simulink model "collection_of_goodies"  (Simulink 5.0)
settings: Solver=ode45  StartTime=0.0  StopTime=10.0  RelTol=1e-3
values from neighbouring files (symbols this model uses):
  c = 4.4*tp/(pi*ts)    [PD_sketch_design.m]
  I = [Ixx,Ixy,Ixz;Iyx,Iyy,Iyz;Izx,Izy,Izz]    [starshotmath.m]
  q0 = [qmatlab(2:4),qmatlab(1)]'    [starshot_DC_KD_setup.m]    (also in starshot_DC_setup.m; temp.m)
  s = tf('s')    [starshot_DC_setup.m]
undefined symbols (not defined in the file or in its folder): a1_T_CMG, a2_T_CMG, a3_T_CMG, AccLim, b1_T_CMG, b2_T_CMG, b3_T_CMG, CFthreshoff, CFthreshon, filt1d, filt1n, filt2d, filt2n, filts1n, filts2d, filts2n, fine, h, h_cos_cmg, h_init, h_sin_cmg, hdmax, hmax, I34, Id, Igm1d, Igm1n, IgmAAFd, invI, invId, Is, Isat, IsatSp, k1_obs, k2_obs, Kt, Kts, lam, Lgm, ls, lt, M34, muE, Ngear, P0, pfd, pfn, q_init, r0, rc_ampl, rc_harm, rc_phase, Rgm, Smin, SmotDrag, spin_init, TachAAFd, TAU_ACS, tr_ampl, tr_harm ... (+8)
libraries: simulink x27, mblibv1 x3, dspinverses x1
(part 2 of 2)

== system collection_of_goodies/Kane Damper wbn is inertial body rate in body axes apply (-Tdamp) to rigid body/Cross1 ==
  A : Inport
  B : Inport  Port=2
  Mux4 : Mux  Inputs=3
  Product{,1..5} (6 alike) : Product  SaturateOnIntegerOverflow=on  InputSameDT=on
  Sum : Sum  Inputs=+-  SaturateOnIntegerOverflow=on  InputSameDT=on
  Sum1 : Sum  Inputs=+-  SaturateOnIntegerOverflow=on  InputSameDT=on
  Sum2 : Sum  Inputs=+-  SaturateOnIntegerOverflow=on  InputSameDT=on
  demux2 : Demux  Outputs=3
  demux3 : Demux  Outputs=3
  AxB : Outport  InitialOutput=0
  wires:
  Mux4/1 -> AxB/1
  Sum2/1 -> Mux4/3
  Sum1/1 -> Mux4/2
  Sum/1 -> Mux4/1
  Product5/1 -> Sum2/2
  Product4/1 -> Sum2/1
  Product3/1 -> Sum1/2
  Product2/1 -> Sum1/1
  Product1/1 -> Sum/2
  Product/1 -> Sum/1
  demux3/1 -> Product5/2, Product2/2
  demux2/2 -> Product5/1, Product/1
  demux3/2 -> Product4/2, Product1/2
  demux2/1 -> Product4/1, Product3/1
  demux3/3 -> Product3/2, Product/2
  demux2/3 -> Product2/1, Product1/1
  B/1 -> demux3/1
  A/1 -> demux2/1

== system collection_of_goodies/Orbit EOM/norm ==
  v : Inport
  Dot Product : simulink/Math Operations/Dot Product
  Math Function : Math  Operator=sqrt
  Saturation : Saturate  UpperLimit=1e20  LowerLimit=1e-10
  |v| : Outport
  wires:
  Saturation/1 -> |v|/1
  Math Function/1 -> Saturation/1
  Dot Product/1 -> Math Function/1
  v/1 -> Dot Product/2, Dot Product/1

== system collection_of_goodies/Propagate Attitude via DCM (not as nice as the quaternion method)/(a*phi)^X ==
  In1 : Inport
  3x3 : simulink/Math Operations/Reshape  OutputDimensionality=Customize  OutputDimensions=[3,3]
  Demux : Demux  Outputs=3
  Gain : Gain  Gain=-1  SaturateOnIntegerOverflow=on
  Gain1 : Gain  Gain=-1  SaturateOnIntegerOverflow=on
  Gain2 : Gain  Gain=-1  SaturateOnIntegerOverflow=on
  Mux : Mux  Inputs=9
  "diag 0 " : Constant  Value=0
  Out1 : Outport
  wires:
  In1/1 -> Demux/1
  3x3/1 -> Out1/1
  "diag 0 "/1 -> Mux/1, Mux/5, Mux/9
  Mux/1 -> 3x3/1
  Demux/3 -> Mux/2, Gain1/1
  Gain/1 -> Mux/3
  Demux/2 -> Gain/1, Mux/7
  Gain1/1 -> Mux/4
  Demux/1 -> Mux/6, Gain2/1
  Gain2/1 -> Mux/8

== system collection_of_goodies/Propagate Attitude via Quaternion/q_normalize ==
  q_in : Inport  PortDimensions=4
  Dot Product : simulink/Math Operations/Dot Product
  Math Function : Math  Operator=sqrt
  Product : Product  Inputs=*/  SaturateOnIntegerOverflow=on  InputSameDT=on
  q_out : Outport
  wires:
  q_in/1 -> Dot Product/1, Dot Product/2, Product/1
  Dot Product/1 -> Math Function/1
  Math Function/1 -> Product/2
  Product/1 -> q_out/1

== system collection_of_goodies/Propagate Attitude via Quaternion/quat_multiply ==
  q_bc : Inport
  q_ab : Inport  Port=2
  Mux : Mux  Inputs=2
  Mux1 : Mux
  qerr1 : Fcn  Expr=u(4)*u(5)+u(3)*u(6)-u(2)*u(7)+u(1)*u(8)
  qerr2 : Fcn  Expr=-u(3)*u(5)+u(4)*u(6)+u(1)*u(7)+u(2)*u(8)
  qerr3 : Fcn  Expr=u(2)*u(5)-u(1)*u(6)+u(4)*u(7)+u(3)*u(8)
  qerr4 : Fcn  Expr=-u(1)*u(5)-u(2)*u(6)-u(3)*u(7)+u(4)*u(8)
  q_ac : Outport
  wires:
  Mux1/1 -> q_ac/1
  qerr4/1 -> Mux1/4
  qerr3/1 -> Mux1/3
  qerr2/1 -> Mux1/2
  qerr1/1 -> Mux1/1
  Mux/1 -> qerr4/1, qerr3/1, qerr2/1, qerr1/1
  q_ab/1 -> Mux/2
  q_bc/1 -> Mux/1

== system collection_of_goodies/Quaternion Integration/q_normalize ==
  q_in : Inport  PortDimensions=4
  Dot Product : simulink/Math Operations/Dot Product
  Math Function : Math  Operator=sqrt
  Product : Product  Inputs=*/  SaturateOnIntegerOverflow=on  InputSameDT=on
  q_out : Outport
  wires:
  q_in/1 -> Dot Product/1, Dot Product/2, Product/1
  Dot Product/1 -> Math Function/1
  Math Function/1 -> Product/2
  Product/1 -> q_out/1

== system collection_of_goodies/Quaternion Integration/qderiv ==
  w : Inport
  q : Inport  Port=2
  Mux : Mux  Inputs=2
  Mux1 : Mux
  qd1 : Fcn  Expr=(u(7)*u(1)-u(6)*u(2)+u(5)*u(3))/2
  qd2 : Fcn  Expr=(u(6)*u(1)+u(7)*u(2)-u(4)*u(3))/2
  qd3 : Fcn  Expr=(-u(5)*u(1)+u(4)*u(2)+u(7)*u(3))/2
  qd4 : Fcn  Expr=(-u(4)*u(1)-u(5)*u(2)-u(6)*u(3))/2
  qd : Outport
  wires:
  w/1 -> Mux/1
  q/1 -> Mux/2
  Mux/1 -> qd1/1, qd2/1, qd3/1, qd4/1
  qd1/1 -> Mux1/1
  qd2/1 -> Mux1/2
  qd3/1 -> Mux1/3
  qd4/1 -> Mux1/4
  Mux1/1 -> qd/1

== system collection_of_goodies/Rigid Body with Momentum Actuators and energy dissipation/Cross ==
  A : Inport
  B : Inport  Port=2
  Mux4 : Mux  Inputs=3
  Product{,1..5} (6 alike) : Product  SaturateOnIntegerOverflow=on  InputSameDT=on
  Sum : Sum  Inputs=+-  SaturateOnIntegerOverflow=on  InputSameDT=on
  Sum1 : Sum  Inputs=+-  SaturateOnIntegerOverflow=on  InputSameDT=on
  Sum2 : Sum  Inputs=+-  SaturateOnIntegerOverflow=on  InputSameDT=on
  demux2 : Demux  Outputs=3
  demux3 : Demux  Outputs=3
  AxB : Outport  InitialOutput=0
  wires:
  Mux4/1 -> AxB/1
  Sum2/1 -> Mux4/3
  Sum1/1 -> Mux4/2
  Sum/1 -> Mux4/1
  Product5/1 -> Sum2/2
  Product4/1 -> Sum2/1
  Product3/1 -> Sum1/2
  Product2/1 -> Sum1/1
  Product1/1 -> Sum/2
  Product/1 -> Sum/1
  demux3/1 -> Product5/2, Product2/2
  demux2/2 -> Product5/1, Product/1
  demux3/2 -> Product4/2, Product1/2
  demux2/1 -> Product4/1, Product3/1
  demux3/3 -> Product3/2, Product/2
  demux2/3 -> Product2/1, Product1/1
  B/1 -> demux3/1
  A/1 -> demux2/1

== system collection_of_goodies/Rigid Body with Momentum Actuators and energy dissipation/Cross1 ==
  A : Inport
  B : Inport  Port=2
  Mux4 : Mux  Inputs=3
  Product{,1..5} (6 alike) : Product  SaturateOnIntegerOverflow=on  InputSameDT=on
  Sum : Sum  Inputs=+-  SaturateOnIntegerOverflow=on  InputSameDT=on
  Sum1 : Sum  Inputs=+-  SaturateOnIntegerOverflow=on  InputSameDT=on
  Sum2 : Sum  Inputs=+-  SaturateOnIntegerOverflow=on  InputSameDT=on
  demux2 : Demux  Outputs=3
  demux3 : Demux  Outputs=3
  AxB : Outport  InitialOutput=0
  wires:
  Mux4/1 -> AxB/1
  Sum2/1 -> Mux4/3
  Sum1/1 -> Mux4/2
  Sum/1 -> Mux4/1
  Product5/1 -> Sum2/2
  Product4/1 -> Sum2/1
  Product3/1 -> Sum1/2
  Product2/1 -> Sum1/1
  Product1/1 -> Sum/2
  Product/1 -> Sum/1
  demux3/1 -> Product5/2, Product2/2
  demux2/2 -> Product5/1, Product/1
  demux3/2 -> Product4/2, Product1/2
  demux2/1 -> Product4/1, Product3/1
  demux3/3 -> Product3/2, Product/2
  demux2/3 -> Product2/1, Product1/1
  B/1 -> demux3/1
  A/1 -> demux2/1

== system collection_of_goodies/Rigid Body with Momentum Actuators and energy dissipation/Quaternion Integration ==
  w_Body : Inport
  Integrator1 : Integrator  InitialCondition=q_init
  q_normalize : Subsystem
  qderiv : Subsystem
  q_I_Body : Outport
  wires:
  qderiv/1(qd) -> Integrator1/1
  Integrator1/1 -> q_normalize/1(q_in)
  q_normalize/1(q_out) -> q_I_Body/1, qderiv/2(q)
  w_Body/1 -> qderiv/1(w)

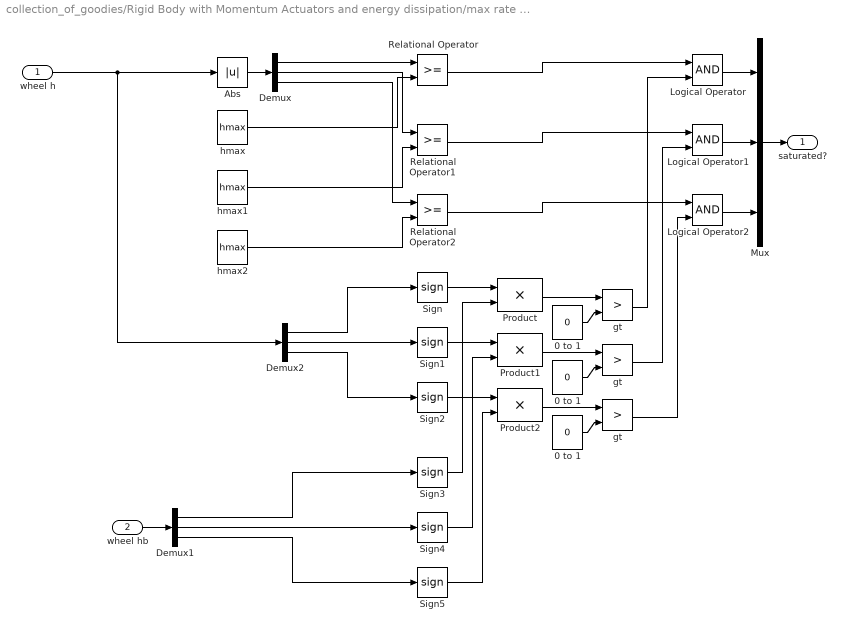
== system collection_of_goodies/Rigid Body with Momentum Actuators and energy dissipation/max rate check ==
  wheel h : Inport
  wheel hb : Inport  Port=2
  0 to 1 : Constant  Value=0  VectorParams1D=off
  "0 to 1 " : Constant  Value=0  VectorParams1D=off
  "0 to 1  " : Constant  Value=0  VectorParams1D=off
  Abs : Abs  SaturateOnIntegerOverflow=on
  Demux : Demux  Outputs=3
  Demux1 : Demux  Outputs=3
  Demux2 : Demux  Outputs=3
  Logical Operator : Logic
  Logical Operator1 : Logic
  Logical Operator2 : Logic
  Mux : Mux  Inputs=3
  Product : Product  SaturateOnIntegerOverflow=on  InputSameDT=on
  Product1 : Product  SaturateOnIntegerOverflow=on  InputSameDT=on
  Product2 : Product  SaturateOnIntegerOverflow=on  InputSameDT=on
  Relational Operator : RelationalOperator  InputSameDT=on
  Relational Operator1 : RelationalOperator  InputSameDT=on
  Relational Operator2 : RelationalOperator  InputSameDT=on
  Sign{,1..5} (6 alike) : Signum
  gt : RelationalOperator  Operator=>  InputSameDT=on
  "gt " : RelationalOperator  Operator=>  InputSameDT=on
  "gt  " : RelationalOperator  Operator=>  InputSameDT=on
  hmax : Constant  Value=hmax  VectorParams1D=off
  hmax1 : Constant  Value=hmax  VectorParams1D=off
  hmax2 : Constant  Value=hmax  VectorParams1D=off
  saturated? : Outport
  wires:
  Abs/1 -> Demux/1
  Demux/1 -> Relational Operator/1
  Demux/2 -> Relational Operator1/1
  Demux/3 -> Relational Operator2/1
  hmax/1 -> Relational Operator/2
  hmax1/1 -> Relational Operator1/2
  hmax2/1 -> Relational Operator2/2
  wheel h/1 -> Abs/1, Demux2/1
  Mux/1 -> saturated?/1
  wheel hb/1 -> Demux1/1
  Demux1/1 -> Sign3/1
  Demux1/2 -> Sign4/1
  Demux1/3 -> Sign5/1
  Sign/1 -> Product/1
  Sign3/1 -> Product/2
  Sign1/1 -> Product1/1
  Sign4/1 -> Product1/2
  Sign2/1 -> Product2/1
  Sign5/1 -> Product2/2
  0 to 1/1 -> gt/2
  Product/1 -> gt/1
  "0 to 1 "/1 -> "gt "/2
  Product1/1 -> "gt "/1
  "0 to 1  "/1 -> "gt  "/2
  Product2/1 -> "gt  "/1
  Logical Operator/1 -> Mux/1
  Logical Operator1/1 -> Mux/2
  Logical Operator2/1 -> Mux/3
  Relational Operator/1 -> Logical Operator/1
  Relational Operator1/1 -> Logical Operator1/1
  Relational Operator2/1 -> Logical Operator2/1
  gt/1 -> Logical Operator/2
  "gt "/1 -> Logical Operator1/2
  "gt  "/1 -> Logical Operator2/2
  Demux2/1 -> Sign/1
  Demux2/2 -> Sign1/1
  Demux2/3 -> Sign2/1

== system collection_of_goodies/SimMechanics embedded h body/cross2 ==
  a : Inport
  b : Inport  Port=2
  Demux : Demux  Outputs=3
  Demux1 : Demux  Outputs=3
  Fcn : Fcn  Expr=-u(3)*u(5)+u(2)*u(6)
  Fcn1 : Fcn  Expr=u(3)*u(4)-u(1)*u(6)
  Fcn2 : Fcn  Expr=-u(2)*u(4)+u(1)*u(5)
  Mux : Mux  Inputs=6
  Mux1 : Mux  Inputs=3
  a x b : Outport
  wires:
  Mux/1 -> Fcn/1, Fcn1/1, Fcn2/1
  Mux1/1 -> a x b/1
  Fcn/1 -> Mux1/1
  Fcn1/1 -> Mux1/2
  Fcn2/1 -> Mux1/3
  Demux/1 -> Mux/1
  Demux/2 -> Mux/2
  Demux/3 -> Mux/3
  a/1 -> Demux/1
  Demux1/1 -> Mux/4
  Demux1/2 -> Mux/5
  Demux1/3 -> Mux/6
  b/1 -> Demux1/1

== system collection_of_goodies/attitude error as axis/angle/axis unit vector ==
  ax_in : Inport
  Constant : Constant  Value=1e-10
  Dot Product : simulink/Math Operations/Dot Product
  Math Function : Math  Operator=sqrt
  Product : Product  Inputs=*/  SaturateOnIntegerOverflow=on  InputSameDT=on
  Switch : Switch  Threshold=1e-10  SaturateOnIntegerOverflow=on  InputSameDT=on
  ax_out : Outport
  wires:
  ax_in/1 -> Dot Product/1, Dot Product/2, Product/1
  Dot Product/1 -> Math Function/1
  Math Function/1 -> Switch/2, Switch/1
  Constant/1 -> Switch/3
  Product/1 -> ax_out/1
  Switch/1 -> Product/2

== system collection_of_goodies/attitude error as axis/angle/q_normalize ==
  q_in : Inport  PortDimensions=4
  Dot Product : simulink/Math Operations/Dot Product
  Math Function : Math  Operator=sqrt
  Product : Product  Inputs=*/  SaturateOnIntegerOverflow=on  InputSameDT=on
  q_out : Outport
  wires:
  q_in/1 -> Dot Product/1, Dot Product/2, Product/1
  Dot Product/1 -> Math Function/1
  Math Function/1 -> Product/2
  Product/1 -> q_out/1

== system collection_of_goodies/attitude error as axis/angle/q_normalize1 ==
  q_in : Inport  PortDimensions=4
  Dot Product : simulink/Math Operations/Dot Product
  Math Function : Math  Operator=sqrt
  Product : Product  Inputs=*/  SaturateOnIntegerOverflow=on  InputSameDT=on
  q_out : Outport
  wires:
  q_in/1 -> Dot Product/1, Dot Product/2, Product/1
  Dot Product/1 -> Math Function/1
  Math Function/1 -> Product/2
  Product/1 -> q_out/1

== system collection_of_goodies/attitude error as axis/angle/q_normalize2 ==
  q_in : Inport  PortDimensions=4
  Dot Product : simulink/Math Operations/Dot Product
  Math Function : Math  Operator=sqrt
  Product : Product  Inputs=*/  SaturateOnIntegerOverflow=on  InputSameDT=on
  q_out : Outport
  wires:
  q_in/1 -> Dot Product/1, Dot Product/2, Product/1
  Dot Product/1 -> Math Function/1
  Math Function/1 -> Product/2
  Product/1 -> q_out/1

== system collection_of_goodies/attitude error as axis/angle/relative_quat1 ==
  q_bc : Inport
  q_ab : Inport  Port=2
  Mux : Mux  Inputs=2
  Mux1 : Mux
  qerr1 : Fcn  Expr=u(4)*u(5)+u(3)*u(6)-u(2)*u(7)+u(1)*u(8)
  qerr2 : Fcn  Expr=-u(3)*u(5)+u(4)*u(6)+u(1)*u(7)+u(2)*u(8)
  qerr3 : Fcn  Expr=u(2)*u(5)-u(1)*u(6)+u(4)*u(7)+u(3)*u(8)
  qerr4 : Fcn  Expr=-u(1)*u(5)-u(2)*u(6)-u(3)*u(7)+u(4)*u(8)
  q_ac : Outport
  wires:
  Mux1/1 -> q_ac/1
  qerr4/1 -> Mux1/4
  qerr3/1 -> Mux1/3
  qerr2/1 -> Mux1/2
  qerr1/1 -> Mux1/1
  Mux/1 -> qerr4/1, qerr3/1, qerr2/1, qerr1/1
  q_ab/1 -> Mux/2
  q_bc/1 -> Mux/1

== system collection_of_goodies/axis/angle to DCM/crs matrix ==
  In1 : Inport
  Constant : Constant  Value=0
  Demux : Demux  Outputs=3
  Gain : Gain  Gain=-1  SaturateOnIntegerOverflow=on
  Gain1 : Gain  Gain=-1  SaturateOnIntegerOverflow=on
  Gain2 : Gain  Gain=-1  SaturateOnIntegerOverflow=on
  Matrix Concatenation : simulink/Math Operations/Matrix Concatenation  numInports=3  catMethod=Horizontal
  Mux : Mux  Inputs=3
  Mux1 : Mux  Inputs=3
  Mux2 : Mux  Inputs=3
  Out1 : Outport
  wires:
  In1/1 -> Demux/1
  Constant/1 -> Mux1/2, Mux/1, Mux2/3
  Demux/3 -> Mux/2, Gain1/1
  Demux/2 -> Gain/1, Mux2/1
  Gain/1 -> Mux/3
  Mux/1 -> Matrix Concatenation/1
  Gain1/1 -> Mux1/1
  Demux/1 -> Mux1/3, Gain2/1
  Mux1/1 -> Matrix Concatenation/2
  Mux2/1 -> Matrix Concatenation/3
  Gain2/1 -> Mux2/2
  Matrix Concatenation/1 -> Out1/1

== system collection_of_goodies/axis/angle to DCM/crs matrix1 ==
  make : Inport
  Constant{,1..5} (6 alike) : Constant  Value=0
  Matrix Concatenation : simulink/Math Operations/Matrix Concatenation  numInports=3  catMethod=Horizontal
  Mux : Mux  Inputs=3
  Mux1 : Mux  Inputs=3
  Mux2 : Mux  Inputs=3
  3x3 : Outport
  wires:
  make/1 -> Mux/1, Mux1/2, Mux2/3
  Mux/1 -> Matrix Concatenation/1
  Mux1/1 -> Matrix Concatenation/2
  Mux2/1 -> Matrix Concatenation/3
  Matrix Concatenation/1 -> 3x3/1
  Constant/1 -> Mux/3
  Constant1/1 -> Mux/2
  Constant2/1 -> Mux1/3
  Constant3/1 -> Mux1/1
  Constant4/1 -> Mux2/2
  Constant5/1 -> Mux2/1

== system collection_of_goodies/compute attitude error/quat_multiply (relative quat) ==
  q_bc : Inport
  q_ab : Inport  Port=2
  Mux : Mux  Inputs=2
  Mux1 : Mux
  qerr1 : Fcn  Expr=u(4)*u(5)+u(3)*u(6)-u(2)*u(7)+u(1)*u(8)
  qerr2 : Fcn  Expr=-u(3)*u(5)+u(4)*u(6)+u(1)*u(7)+u(2)*u(8)
  qerr3 : Fcn  Expr=u(2)*u(5)-u(1)*u(6)+u(4)*u(7)+u(3)*u(8)
  qerr4 : Fcn  Expr=-u(1)*u(5)-u(2)*u(6)-u(3)*u(7)+u(4)*u(8)
  q_ac : Outport
  wires:
  Mux1/1 -> q_ac/1
  qerr4/1 -> Mux1/4
  qerr3/1 -> Mux1/3
  qerr2/1 -> Mux1/2
  qerr1/1 -> Mux1/1
  Mux/1 -> qerr4/1, qerr3/1, qerr2/1, qerr1/1
  q_ab/1 -> Mux/2
  q_bc/1 -> Mux/1

== system collection_of_goodies/quat to DCM/Subsystem ==
  In1 : Inport
  3x3 : simulink/Math Operations/Reshape  OutputDimensionality=Customize  OutputDimensions=[3,3]
  Demux : Demux  Outputs=3
  Gain : Gain  Gain=-1  SaturateOnIntegerOverflow=on
  Gain1 : Gain  Gain=-1  SaturateOnIntegerOverflow=on
  Gain2 : Gain  Gain=-1  SaturateOnIntegerOverflow=on
  Mux : Mux  Inputs=9
  "diag 0 " : Constant  Value=0
  Out1 : Outport
  wires:
  In1/1 -> Demux/1
  3x3/1 -> Out1/1
  "diag 0 "/1 -> Mux/1, Mux/5, Mux/9
  Mux/1 -> 3x3/1
  Demux/3 -> Mux/2, Gain1/1
  Gain/1 -> Mux/3
  Demux/2 -> Gain/1, Mux/7
  Gain1/1 -> Mux/4
  Demux/1 -> Mux/6, Gain2/1
  Gain2/1 -> Mux/8

== system collection_of_goodies/rigid body/Cross1 ==
  A : Inport  PortDimensions=3
  B : Inport  Port=2  PortDimensions=3
  Mux4 : Mux  Inputs=3
  Product{,1..5} (6 alike) : Product  SaturateOnIntegerOverflow=on  InputSameDT=on
  Sum : Sum  Inputs=+-  SaturateOnIntegerOverflow=on  InputSameDT=on
  Sum1 : Sum  Inputs=+-  SaturateOnIntegerOverflow=on  InputSameDT=on
  Sum2 : Sum  Inputs=+-  SaturateOnIntegerOverflow=on  InputSameDT=on
  demux2 : Demux  Outputs=3
  demux3 : Demux  Outputs=3
  AxB : Outport  InitialOutput=0
  wires:
  Mux4/1 -> AxB/1
  Sum2/1 -> Mux4/3
  Sum1/1 -> Mux4/2
  Sum/1 -> Mux4/1
  Product5/1 -> Sum2/2
  Product4/1 -> Sum2/1
  Product3/1 -> Sum1/2
  Product2/1 -> Sum1/1
  Product1/1 -> Sum/2
  Product/1 -> Sum/1
  demux3/1 -> Product5/2, Product2/2
  demux2/2 -> Product5/1, Product/1
  demux3/2 -> Product4/2, Product1/2
  demux2/1 -> Product4/1, Product3/1
  demux3/3 -> Product3/2, Product/2
  demux2/3 -> Product2/1, Product1/1
  B/1 -> demux3/1
  A/1 -> demux2/1

== system collection_of_goodies/AttitudeObserver/AttError/qconjMult ==
  q_cmd : Inport
  q_est : Inport  Port=2
  Mux : Mux  Inputs=2
  Mux1 : Mux
  qerr1 : Fcn  Expr=-u(4)*u(5)-u(3)*u(6)+u(2)*u(7)+u(1)*u(8)
  qerr2 : Fcn  Expr=u(3)*u(5)-u(4)*u(6)-u(1)*u(7)+u(2)*u(8)
  qerr3 : Fcn  Expr=-u(2)*u(5)+u(1)*u(6)-u(4)*u(7)+u(3)*u(8)
  qerr4 : Fcn  Expr=u(1)*u(5)+u(2)*u(6)+u(3)*u(7)+u(4)*u(8)
  q_err : Outport
  wires:
  q_cmd/1 -> Mux/1
  q_est/1 -> Mux/2
  Mux/1 -> qerr1/1, qerr2/1, qerr3/1, qerr4/1
  qerr1/1 -> Mux1/1
  qerr2/1 -> Mux1/2
  qerr3/1 -> Mux1/3
  qerr4/1 -> Mux1/4
  Mux1/1 -> q_err/1

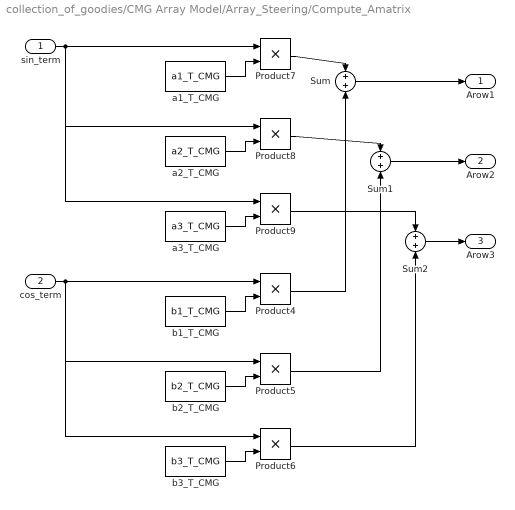
== system collection_of_goodies/CMG Array Model/Array_Steering/Compute_Amatrix ==
  sin_term : Inport  PortDimensions=6
  cos_term : Inport  Port=2  PortDimensions=6
  Product{4..9} (6 alike) : Product  SaturateOnIntegerOverflow=on  InputSameDT=on
  Sum : Sum  SaturateOnIntegerOverflow=on  InputSameDT=on
  Sum1 : Sum  SaturateOnIntegerOverflow=on  InputSameDT=on
  Sum2 : Sum  SaturateOnIntegerOverflow=on  InputSameDT=on
  a1_T_CMG : Constant  Value=a1_T_CMG
  a2_T_CMG : Constant  Value=a2_T_CMG
  a3_T_CMG : Constant  Value=a3_T_CMG
  b1_T_CMG : Constant  Value=b1_T_CMG
  b2_T_CMG : Constant  Value=b2_T_CMG
  b3_T_CMG : Constant  Value=b3_T_CMG
  Arow1 : Outport
  Arow2 : Outport  Port=2
  Arow3 : Outport  Port=3
  wires:
  Sum/1 -> Arow1/1
  Sum1/1 -> Arow2/1
  Sum2/1 -> Arow3/1
  Product6/1 -> Sum2/2
  Product9/1 -> Sum2/1
  Product5/1 -> Sum1/2
  Product8/1 -> Sum1/1
  Product4/1 -> Sum/2
  Product7/1 -> Sum/1
  a3_T_CMG/1 -> Product9/2
  sin_term/1 -> Product9/1, Product8/1, Product7/1
  a2_T_CMG/1 -> Product8/2
  a1_T_CMG/1 -> Product7/2
  b3_T_CMG/1 -> Product6/2
  cos_term/1 -> Product6/1, Product5/1, Product4/1
  b2_T_CMG/1 -> Product5/2
  b1_T_CMG/1 -> Product4/2

== system collection_of_goodies/CMG Gimbal Control System/Actuator/Bemf Phases ==
  In : Inport
  Angle : Inport  Port=2
  Elect Freq : Gain  Gain=12  SaturateOnIntegerOverflow=on
  Mux : Mux  Inputs=2
  Product2 : Product  SaturateOnIntegerOverflow=on  InputSameDT=on
  Product3 : Product  SaturateOnIntegerOverflow=on  InputSameDT=on
  Trigonometric Function : Trigonometry  Orientation=up
  Trigonometric Function1 : Trigonometry  Orientation=up  Operator=cos
  Out : Outport  InitialOutput=0
  wires:
  Mux/1 -> Out/1
  Angle/1 -> Elect Freq/1
  In/1 -> Product2/1, Product3/1
  Trigonometric Function1/1 -> Product3/2
  Trigonometric Function/1 -> Product2/2
  Product2/1 -> Mux/1
  Product3/1 -> Mux/2
  Elect Freq/1 -> Trigonometric Function1/1, Trigonometric Function/1

== system collection_of_goodies/CMG Gimbal Control System/Actuator/Braking ==
  Back EMF : Inport
  Driver Voltage : Inport  Port=2
  Current : Inport  Port=3
  Terminal Voltage : Outport  InitialOutput=0
  wires:
  Driver Voltage/1 -> Terminal Voltage/1

== system collection_of_goodies/CMG Gimbal Control System/Actuator/Motor Coil ==
  Back EMF : Inport
  Terminal Voltage : Inport  Port=2
  Demux1 : Demux  Outputs=2
  Demux2 : Demux  Outputs=2
  Gimbal Motor Coil : TransferFcn  Denominator=[Lgm Rgm]
  Gimbal Motor Coil1 : TransferFcn  Denominator=[Lgm Rgm]
  Mux : Mux  Inputs=2
  Sum4 : Sum  Inputs=-+  SaturateOnIntegerOverflow=on  InputSameDT=on
  Sum6 : Sum  Inputs=-+  SaturateOnIntegerOverflow=on  InputSameDT=on
  Current : Outport  InitialOutput=0
  wires:
  Back EMF/1 -> Demux1/1
  Terminal Voltage/1 -> Demux2/1
  Sum4/1 -> Gimbal Motor Coil/1
  Sum6/1 -> Gimbal Motor Coil1/1
  Mux/1 -> Current/1
  Demux2/2 -> Sum6/2
  Demux2/1 -> Sum4/2
  Demux1/2 -> Sum6/1
  Demux1/1 -> Sum4/1
  Gimbal Motor Coil/1 -> Mux/1
  Gimbal Motor Coil1/1 -> Mux/2

== system collection_of_goodies/CMG Gimbal Control System/Actuator/Motor Ripple ==
  note: Ripple
      | Factor
  note: Cogging
      | Torque
      | (terms)
  Torque In : Inport
  Motor Angle : Inport  Port=2
  Amplitude : Constant  Orientation=up  Value=rc_ampl
  Demux : Demux  Outputs=[4 5]
  Harmonic : Constant  Orientation=up  Value=rc_harm
  Phase : Constant  Orientation=down  Value=rc_phase
  Product : Product  SaturateOnIntegerOverflow=on  InputSameDT=on
  Product1 : Product  SaturateOnIntegerOverflow=on  InputSameDT=on
  Product2 : Product  SaturateOnIntegerOverflow=on  InputSameDT=on
  Sum : Sum  Inputs=++|  SaturateOnIntegerOverflow=on  InputSameDT=on
  Sum3 : Sum  Inputs=+  SaturateOnIntegerOverflow=on  InputSameDT=on
  Sum4 : Sum  Inputs=+  SaturateOnIntegerOverflow=on  InputSameDT=on
  Sum5 : Sum  SaturateOnIntegerOverflow=on  InputSameDT=on
  Trigonometric Function : Trigonometry  Operator=cos
  Torque Ripple : Outport  InitialOutput=0
  wires:
  Product/1 -> Trigonometric Function/1
  Trigonometric Function/1 -> Product2/1
  Product2/1 -> Demux/1
  Harmonic/1 -> Product/2
  Amplitude/1 -> Product2/2
  Demux/1 -> Sum3/1
  Demux/2 -> Sum4/1
  Sum3/1 -> Sum5/1
  Sum5/1 -> Torque Ripple/1
  Product1/1 -> Sum5/2
  Sum4/1 -> Product1/1
  Torque In/1 -> Product1/2
  Motor Angle/1 -> Sum/2
  Sum/1 -> Product/1
  Phase/1 -> Sum/1

== system collection_of_goodies/CMG Gimbal Control System/Actuator/Torque Phases ==
  In : Inport
  Angle : Inport  Port=2
  Demux1 : Demux  Outputs=2
  Elect Freq : Gain  Gain=12  SaturateOnIntegerOverflow=on
  Product2 : Product  SaturateOnIntegerOverflow=on  InputSameDT=on
  Product3 : Product  SaturateOnIntegerOverflow=on  InputSameDT=on
  Sum5 : Sum  SaturateOnIntegerOverflow=on  InputSameDT=on
  Trigonometric Function : Trigonometry  Orientation=up
  Trigonometric Function1 : Trigonometry  Orientation=up  Operator=cos
  Out : Outport  InitialOutput=0
  wires:
  Elect Freq/1 -> Trigonometric Function/1, Trigonometric Function1/1
  Trigonometric Function/1 -> Product2/2
  Trigonometric Function1/1 -> Product3/2
  Angle/1 -> Elect Freq/1
  Product2/1 -> Sum5/1
  Product3/1 -> Sum5/2
  Sum5/1 -> Out/1
  Demux1/1 -> Product2/1
  Demux1/2 -> Product3/1
  In/1 -> Demux1/1

== system collection_of_goodies/CMG Gimbal Control System/Control/Rate Feedback ==
  Coarse/Fine : Inport
  Abs : Abs  SaturateOnIntegerOverflow=on
  Demux1 : Demux  Outputs=2
  Fine Gain Correction : Gain  Gain=1/fine  SaturateOnIntegerOverflow=on
  Relay : Relay  OnSwitchValue=CFthreshon  OffSwitchValue=CFthreshoff
  Switch : Switch  Threshold=.5  SaturateOnIntegerOverflow=on  InputSameDT=on
  Composite : Outport  InitialOutput=0
  wires:
  Coarse/Fine/1 -> Demux1/1
  Demux1/2 -> Fine Gain Correction/1
  Fine Gain Correction/1 -> Switch/3
  Relay/1 -> Switch/2
  Demux1/1 -> Switch/1, Abs/1
  Abs/1 -> Relay/1
  Switch/1 -> Composite/1

== system collection_of_goodies/CMG Gimbal Control System/Control/Rate Loop Compensation ==
  Rate Error : Inport
  "\"Bi-Quad\"" : TransferFcn  Numerator=filt1n  Denominator=filt1d
  Integrator : Integrator  LimitOutput=on  UpperSaturationLimit=Isat  LowerSaturationLimit=-Isat
  Lead/Lag : TransferFcn  Numerator=filt2n  Denominator=filt2d
  Current Cmd : Outport  InitialOutput=0
  wires:
  "\"Bi-Quad\""/1 -> Lead/Lag/1
  Rate Error/1 -> "\"Bi-Quad\""/1
  Integrator/1 -> Current Cmd/1
  Lead/Lag/1 -> Integrator/1

== system collection_of_goodies/CMG Gimbal Control System/Control/Resolver Logic ==
  Resolver : Inport
  Demux1 : Demux
  Gain1 : Gain  Gain=1/32  SaturateOnIntegerOverflow=on
  Trigonometric Function : Trigonometry  Operator=atan2
  Trigonometric Function1 : Trigonometry  Operator=atan2
  Measured Shaft Angle : Outport  InitialOutput=0
  wires:
  Resolver/1 -> Demux1/1
  Demux1/1 -> Trigonometric Function/1
  Demux1/2 -> Trigonometric Function/2
  Demux1/3 -> Trigonometric Function1/1
  Demux1/4 -> Trigonometric Function1/2
  Trigonometric Function1/1 -> Measured Shaft Angle/1
  Trigonometric Function/1 -> Gain1/1

== system collection_of_goodies/CMG Gimbal Control System/Control/SpeedQuant ==
  note: Qspeed in sec/rad to emulate timing of one rev
  In : Inport
  Math Function : Math  Operator=reciprocal
  Math Function1 : Math  Operator=reciprocal
  Qspeed : Quantizer  QuantizationInterval=Qspeed
  SpeedMin : Saturate  UpperLimit=inf  LowerLimit=Smin
  Out : Outport  InitialOutput=0
  wires:
  Math Function/1 -> Qspeed/1
  Math Function1/1 -> Out/1
  Qspeed/1 -> Math Function1/1
  In/1 -> SpeedMin/1
  SpeedMin/1 -> Math Function/1

== system collection_of_goodies/CMG Gimbal Control System/Control/Spin Loop Compensation ==
  Rate Error : Inport
  Integrator : Integrator  InitialCondition=spin_init  LimitOutput=on  UpperSaturationLimit=IsatSp  LowerSaturationLimit=-IsatSp
  Lead/Lag : TransferFcn  Numerator=filts2n  Denominator=filts2d
  filts1n : Gain  Gain=filts1n  SaturateOnIntegerOverflow=on
  Current Cmd : Outport  InitialOutput=0
  wires:
  Rate Error/1 -> Lead/Lag/1
  Lead/Lag/1 -> filts1n/1
  filts1n/1 -> Integrator/1
  Integrator/1 -> Current Cmd/1

== system collection_of_goodies/CMG Gimbal Control System/Control/TorqueComm ==
  Current Command : Inport
  Meas Shaft Angle : Inport  Port=2
  Gain1 : Gain  Gain=12  SaturateOnIntegerOverflow=on
  Mux : Mux  Inputs=2
  Product : Product  SaturateOnIntegerOverflow=on  InputSameDT=on
  Product1 : Product  SaturateOnIntegerOverflow=on  InputSameDT=on
  Trigonometric Function : Trigonometry
  Trigonometric Function1 : Trigonometry  Operator=cos
  Current Cmds : Outport  InitialOutput=0
  wires:
  Mux/1 -> Current Cmds/1
  Current Command/1 -> Product/1, Product1/1
  Meas Shaft Angle/1 -> Gain1/1
  Gain1/1 -> Trigonometric Function/1, Trigonometric Function1/1
  Trigonometric Function/1 -> Product/2
  Trigonometric Function1/1 -> Product1/2
  Product/1 -> Mux/1
  Product1/1 -> Mux/2

== system collection_of_goodies/CMG Gimbal Control System/Drive/Current Loop 1 ==
  CurrentCmd : Inport
  Current : Inport  Orientation=left  Port=2
  AAF : TransferFcn  Orientation=left  Denominator=IgmAAFd
  Current Loop Compensation : TransferFcn  Numerator=Igm1n  Denominator=Igm1d
  PWM : Gain  SaturateOnIntegerOverflow=on
  Sum : Sum  Inputs=+-  SaturateOnIntegerOverflow=on  InputSameDT=on
  Vbus : Saturate  UpperLimit=Vsat  LowerLimit=-Vsat
  VcoilQuant : Quantizer  QuantizationInterval=Qvcoil
  Vanalog : Outport  InitialOutput=0
  CurSense : Outport  Orientation=left  Port=2  InitialOutput=0
  wires:
  CurrentCmd/1 -> Sum/1
  VcoilQuant/1 -> Vanalog/1
  Vbus/1 -> VcoilQuant/1
  Current/1 -> AAF/1
  PWM/1 -> Vbus/1
  Current Loop Compensation/1 -> PWM/1
  AAF/1 -> Sum/2, CurSense/1
  Sum/1 -> Current Loop Compensation/1

== system collection_of_goodies/CMG Gimbal Control System/Drive/Current Loop 2 ==
  CurrentCmd : Inport
  Current : Inport  Orientation=left  Port=2
  AAF : TransferFcn  Orientation=left  Denominator=IgmAAFd
  Current Loop Compensation : TransferFcn  Numerator=Igm1n  Denominator=Igm1d
  PWM : Gain  SaturateOnIntegerOverflow=on
  Sum : Sum  Inputs=+-  SaturateOnIntegerOverflow=on  InputSameDT=on
  Vbus : Saturate  UpperLimit=Vsat  LowerLimit=-Vsat
  VcoilQuant : Quantizer  QuantizationInterval=Qvcoil
  Vanalog : Outport  InitialOutput=0
  CurSense : Outport  Orientation=left  Port=2  InitialOutput=0
  wires:
  Sum/1 -> Current Loop Compensation/1
  AAF/1 -> CurSense/1, Sum/2
  Current Loop Compensation/1 -> PWM/1
  PWM/1 -> Vbus/1
  Current/1 -> AAF/1
  Vbus/1 -> VcoilQuant/1
  VcoilQuant/1 -> Vanalog/1
  CurrentCmd/1 -> Sum/1

== system collection_of_goodies/CMG Gimbal Control System/Sensor/Resolvers ==
  Truth Angle : Inport
  32x : Gain  Gain=32  SaturateOnIntegerOverflow=on
  AAF{,1..3} (4 alike) : TransferFcn  Denominator=[1/(2*pi*250) 1]
  Mux4 : Mux
  Trigonometric Function : Trigonometry
  Trigonometric Function1 : Trigonometry  Operator=cos
  Trigonometric Function2 : Trigonometry
  Trigonometric Function3 : Trigonometry  Operator=cos
  Resolver Out : Outport  InitialOutput=0
  wires:
  Mux4/1 -> Resolver Out/1
  AAF/1 -> Mux4/1
  Trigonometric Function/1 -> AAF/1
  32x/1 -> Trigonometric Function/1, Trigonometric Function1/1
  Truth Angle/1 -> 32x/1, Trigonometric Function2/1, Trigonometric Function3/1
  Trigonometric Function1/1 -> AAF1/1
  Trigonometric Function2/1 -> AAF2/1
  Trigonometric Function3/1 -> AAF3/1
  AAF1/1 -> Mux4/2
  AAF2/1 -> Mux4/3
  AAF3/1 -> Mux4/4

== system collection_of_goodies/CMG Gimbal Control System/Sensor/Tach Phases ==
  note: Add model of each phase based on truth angle,
      | then mux to one per Tach Commutation input
  TachComm : Inport
  Rate : Inport  Port=2
  Truth Angle : Inport  Port=3
  Meas Rate : Outport  InitialOutput=0
  wires:
  Rate/1 -> Meas Rate/1

== system collection_of_goodies/CMG Gimbal Control System/Sensor/Tach Ripple ==
  note: Ripple
      | Factor
  note: Ripple
      | Term
  Rate In : Inport
  Motor Angle : Inport  Port=2
  Amplitude : Constant  Orientation=up  Value=tr_ampl
  Demux : Demux  Outputs=[2 8]
  Harmonic : Constant  Orientation=up  Value=tr_harm
  Phase : Constant  Orientation=down  Value=tr_phase
  Product : Product  SaturateOnIntegerOverflow=on  InputSameDT=on
  Product1 : Product  SaturateOnIntegerOverflow=on  InputSameDT=on
  Product2 : Product  SaturateOnIntegerOverflow=on  InputSameDT=on
  Sum : Sum  Inputs=++|  SaturateOnIntegerOverflow=on  InputSameDT=on
  Sum3 : Sum  Inputs=+  SaturateOnIntegerOverflow=on  InputSameDT=on
  Sum4 : Sum  Inputs=+  SaturateOnIntegerOverflow=on  InputSameDT=on
  Sum5 : Sum  SaturateOnIntegerOverflow=on  InputSameDT=on
  Trigonometric Function : Trigonometry  Operator=cos
  Tach Ripple : Outport  InitialOutput=0
  wires:
  Sum5/1 -> Tach Ripple/1
  Product1/1 -> Sum5/2
  Demux/2 -> Sum4/1
  Demux/1 -> Sum3/1
  Amplitude/1 -> Product2/2
  Harmonic/1 -> Product/2
  Product2/1 -> Demux/1
  Trigonometric Function/1 -> Product2/1
  Product/1 -> Trigonometric Function/1
  Rate In/1 -> Product1/2
  Sum4/1 -> Product1/1
  Sum3/1 -> Sum5/1
  Phase/1 -> Sum/1
  Motor Angle/1 -> Sum/2
  Sum/1 -> Product/1

== system collection_of_goodies/Rigid Body with Momentum Actuators and energy dissipation/Quaternion Integration/q_normalize ==
  q_in : Inport  PortDimensions=4
  Dot Product : simulink/Math Operations/Dot Product
  Math Function : Math  Operator=sqrt
  Product : Product  Inputs=*/  SaturateOnIntegerOverflow=on  InputSameDT=on
  q_out : Outport
  wires:
  q_in/1 -> Dot Product/1, Dot Product/2, Product/1
  Dot Product/1 -> Math Function/1
  Math Function/1 -> Product/2
  Product/1 -> q_out/1

== system collection_of_goodies/Rigid Body with Momentum Actuators and energy dissipation/Quaternion Integration/qderiv ==
  w : Inport
  q : Inport  Port=2
  Mux : Mux  Inputs=2
  Mux1 : Mux
  qd1 : Fcn  Expr=(u(7)*u(1)-u(6)*u(2)+u(5)*u(3))/2
  qd2 : Fcn  Expr=(u(6)*u(1)+u(7)*u(2)-u(4)*u(3))/2
  qd3 : Fcn  Expr=(-u(5)*u(1)+u(4)*u(2)+u(7)*u(3))/2
  qd4 : Fcn  Expr=(-u(4)*u(1)-u(5)*u(2)-u(6)*u(3))/2
  qd : Outport
  wires:
  w/1 -> Mux/1
  q/1 -> Mux/2
  Mux/1 -> qd1/1, qd2/1, qd3/1, qd4/1
  qd1/1 -> Mux1/1
  qd2/1 -> Mux1/2
  qd3/1 -> Mux1/3
  qd4/1 -> Mux1/4
  Mux1/1 -> qd/1
